simulink model "c2_4zhuangtaiguance"  (R2019b)
settings: Solver=VariableStepAuto  StartTime=0.0  StopTime=70  RelTol=1e-3
settings Model: Creator=MAY  LastModifiedBy=wy151
settings DataIOCC: ReturnWorkspaceOutputs=off
settings OptimizationCC: LifeSpan=inf
settings DebuggingCC: SFExecutionAtInitializationDiag=none  ArithmeticOperatorsInVariantConditions=warning
settings SFSimCC: SimUseLocalCustomCode=off  CustomCodeUndefinedFunction=UseInterfaceOnly
settings RTWCC: RTWUseLocalCustomCode=off
settings CodeAppCC: StateflowObjectComments=on

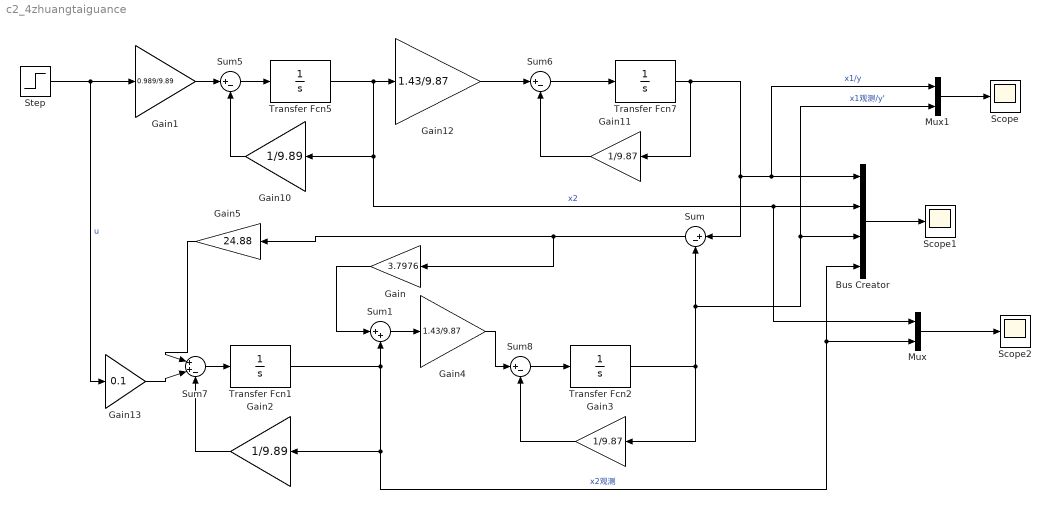
== system c2_4zhuangtaiguance ==
  Bus Creator : BusCreator  Inputs=4
  Gain : Gain  Gain=3.7976
  Gain1 : Gain  Gain=0.989/9.89
  Gain10 : Gain  Gain=1/9.89
  Gain11 : Gain  Gain=1/9.87
  Gain12 : Gain  Gain=1.43/9.87
  Gain13 : Gain  Gain=0.1
  Gain2 : Gain  Gain=1/9.89
  Gain3 : Gain  Gain=1/9.87
  Gain4 : Gain  Gain=1.43/9.87
  Gain5 : Gain  Gain=24.88
  Mux : Mux  Inputs=2
  Mux1 : Mux  Inputs=2
  Scope : Scope
  Scope1 : Scope
  Scope2 : Scope
  Step : Step  SampleTime=0
  Sum{,5..6,8} (4 alike) : Sum  Inputs=|+-
  Sum1 : Sum  Inputs=|++
  Sum7 : Sum  Inputs=|++-
  Transfer Fcn{1..2,5,7} (4 alike) : TransferFcn  Denominator=[1 0]
  wires:
  Transfer Fcn5/1 -> Gain12/1, Gain10/1, Bus Creator/2, Mux/1  "x2"
  Transfer Fcn7/1 -> Sum/1, Bus Creator/1, Mux1/1, Gain11/1  "x1/y"
  Step/1 -> Gain13/1, Gain1/1  "u"
  Bus Creator/1 -> Scope1/1
  Sum/1 -> Gain5/1, Gain/1
  Gain/1 -> Sum1/1
  Gain5/1 -> Sum7/1
  Transfer Fcn1/1 -> Gain2/1, Mux/2, Bus Creator/4, Sum1/2  "x2观测"
  Transfer Fcn2/1 -> Gain3/1, Sum/2, Bus Creator/3, Mux1/2  "x1观测/y'"
  Gain1/1 -> Sum5/1
  Sum5/1 -> Transfer Fcn5/1
  Gain10/1 -> Sum5/2
  Gain12/1 -> Sum6/1
  Sum6/1 -> Transfer Fcn7/1
  Gain11/1 -> Sum6/2
  Sum7/1 -> Transfer Fcn1/1
  Gain3/1 -> Sum8/2
  Sum8/1 -> Transfer Fcn2/1
  Sum1/1 -> Gain4/1
  Gain4/1 -> Sum8/1
  Gain2/1 -> Sum7/3
  Gain13/1 -> Sum7/2
  Mux/1 -> Scope2/1
  Mux1/1 -> Scope/1
